simulink model "Pump_system_008"  (R2020a)
settings: Solver=VariableStepAuto  StartTime=0.0  StopTime=1000  MaxStep=0.5  RelTol=1e-3  AbsTol=1e-4
libraries: subsea_lib x65, nesl_utility x44
(part 2 of 2)

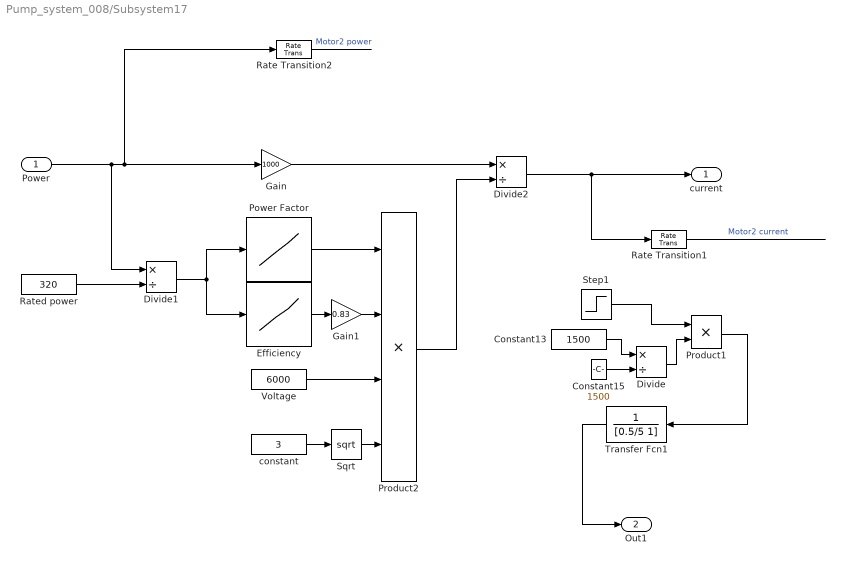
== system Pump_system_008/Subsystem17 ==
  Power : Inport
  Constant13 : Constant  Value=1500
  Constant15 : Constant  Value=1500
  Divide : Product  Inputs=*/
  Divide1 : Product  Inputs=*/
  Divide2 : Product  Inputs=*/
  Efficiency : Lookup_n-D  NumberOfTableDimensions=1  BreakpointsForDimension1=[0 0.05 0.25 0.5 0.75 1]  BreakpointsForDimension2=[1:3]  Table=[0 0.3 0.85 0.92 0.93 0.94]  InternalRulePriority=Speed  RndMeth=Simplest  InputSameDT=on
  Gain : Gain  Gain=1000
  Gain1 : Gain  Gain=0.83
  Power Factor : Lookup_n-D  NumberOfTableDimensions=1  BreakpointsForDimension1=[0 0.05 0.25 0.5 0.75 1]  BreakpointsForDimension2=[1:3]  Table=[0 0.3 0.7 0.83 0.85 0.87]  InternalRulePriority=Speed  RndMeth=Simplest  InputSameDT=on
  Product1 : Product
  Product2 : Product  Inputs=4
  Rate Transition1 : RateTransition  OutPortSampleTime=1
  Rate Transition2 : RateTransition  OutPortSampleTime=1
  Rated power : Constant  Value=320
  Sqrt : Sqrt  SaturateOnIntegerOverflow=on
  Step1 : Step  Time=0.1  SampleTime=0
  Transfer Fcn1 : TransferFcn  Denominator=[0.5/5 1]
  Voltage : Constant  Value=6000
  constant : Constant  Value=3
  current : Outport
  Out1 : Outport  Port=2
  wires:
  Gain/1 -> Divide2/1
  Product2/1 -> Divide2/2
  Power Factor/1 -> Product2/1
  Efficiency/1 -> Gain1/1
  Sqrt/1 -> Product2/4
  constant/1 -> Sqrt/1
  Voltage/1 -> Product2/3
  Divide1/1 -> Power Factor/1, Efficiency/1
  Rated power/1 -> Divide1/2
  Power/1 -> Rate Transition2/1, Gain/1, Divide1/1
  Step1/1 -> Product1/1
  Transfer Fcn1/1 -> Out1/1
  Constant15/1 -> Divide/2
  Divide/1 -> Product1/2
  Product1/1 -> Transfer Fcn1/1
  Constant13/1 -> Divide/1
  Rate Transition2/1 -> ?  "Motor2 power"
  Rate Transition1/1 -> ?  "Motor2 current"
  Divide2/1 -> Rate Transition1/1, current/1
  Gain1/1 -> Product2/2

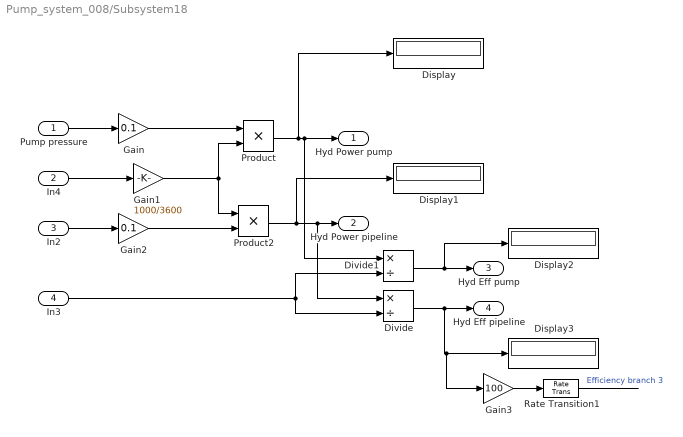
== system Pump_system_008/Subsystem18 ==
  Pump pressure : Inport
  In4 : Inport  Port=2
  In2 : Inport  Port=3
  In3 : Inport  Port=4
  Display{,1..3} (4 alike) : Display
      settings: Decimation=2
  Divide : Product  Inputs=*/
  Divide1 : Product  Inputs=*/
  Gain : Gain  Gain=0.1
  Gain1 : Gain  Gain=1000/3600
  Gain2 : Gain  Gain=0.1
  Gain3 : Gain  Gain=100
  Product : Product
  Product2 : Product
  Rate Transition1 : RateTransition  OutPortSampleTime=1
  Hyd Power pump : Outport
  Hyd Power pipeline : Outport  Port=2
  Hyd Eff pump : Outport  Port=3
  Hyd Eff pipeline : Outport  Port=4
  wires:
  Divide/1 -> Hyd Eff pipeline/1, Gain3/1, Display3/1
  Divide1/1 -> Hyd Eff pump/1, Display2/1
  Product2/1 -> Display1/1, Hyd Power pipeline/1, Divide/1
  Gain2/1 -> Product2/2
  Gain1/1 -> Product2/1, Product/2
  Gain/1 -> Product/1
  Pump pressure/1 -> Gain/1
  In3/1 -> Divide/2, Divide1/2
  In4/1 -> Gain1/1
  Product/1 -> Hyd Power pump/1, Divide1/1, Display/1
  In2/1 -> Gain2/1
  Gain3/1 -> Rate Transition1/1
  Rate Transition1/1 -> ?  "Efficiency branch 3"

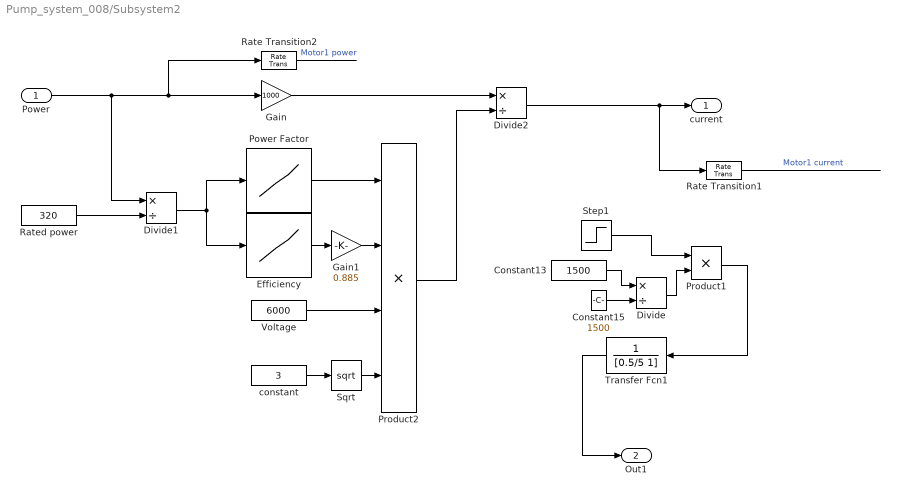
== system Pump_system_008/Subsystem2 ==
  Power : Inport
  Constant13 : Constant  Value=1500
  Constant15 : Constant  Value=1500
  Divide : Product  Inputs=*/
  Divide1 : Product  Inputs=*/
  Divide2 : Product  Inputs=*/
  Efficiency : Lookup_n-D  NumberOfTableDimensions=1  BreakpointsForDimension1=[0 0.05 0.25 0.5 0.75 1]  BreakpointsForDimension2=[1:3]  Table=[0 0.3 0.85 0.92 0.93 0.94]  InternalRulePriority=Speed  RndMeth=Simplest  InputSameDT=on
  Gain : Gain  Gain=1000
  Gain1 : Gain  Gain=0.885
  Power Factor : Lookup_n-D  NumberOfTableDimensions=1  BreakpointsForDimension1=[0 0.05 0.25 0.5 0.75 1]  BreakpointsForDimension2=[1:3]  Table=[0 0.3 0.7 0.85 0.88 0.92]  InternalRulePriority=Speed  RndMeth=Simplest  InputSameDT=on
  Product1 : Product
  Product2 : Product  Inputs=4
  Rate Transition1 : RateTransition  OutPortSampleTime=1
  Rate Transition2 : RateTransition  OutPortSampleTime=1
  Rated power : Constant  Value=320
  Sqrt : Sqrt  SaturateOnIntegerOverflow=on
  Step1 : Step  Time=0.1  SampleTime=0
  Transfer Fcn1 : TransferFcn  Denominator=[0.5/5 1]
  Voltage : Constant  Value=6000
  constant : Constant  Value=3
  current : Outport
  Out1 : Outport  Port=2
  wires:
  Constant13/1 -> Divide/1
  Product1/1 -> Transfer Fcn1/1
  Divide/1 -> Product1/2
  Constant15/1 -> Divide/2
  Transfer Fcn1/1 -> Out1/1
  Step1/1 -> Product1/1
  Power/1 -> Divide1/1, Rate Transition2/1, Gain/1
  Rated power/1 -> Divide1/2
  Divide1/1 -> Efficiency/1, Power Factor/1
  Voltage/1 -> Product2/3
  constant/1 -> Sqrt/1
  Sqrt/1 -> Product2/4
  Efficiency/1 -> Gain1/1
  Power Factor/1 -> Product2/1
  Product2/1 -> Divide2/2
  Gain/1 -> Divide2/1
  Divide2/1 -> Rate Transition1/1, current/1
  Rate Transition1/1 -> ?  "Motor1 current"
  Rate Transition2/1 -> ?  "Motor1 power"
  Gain1/1 -> Product2/2

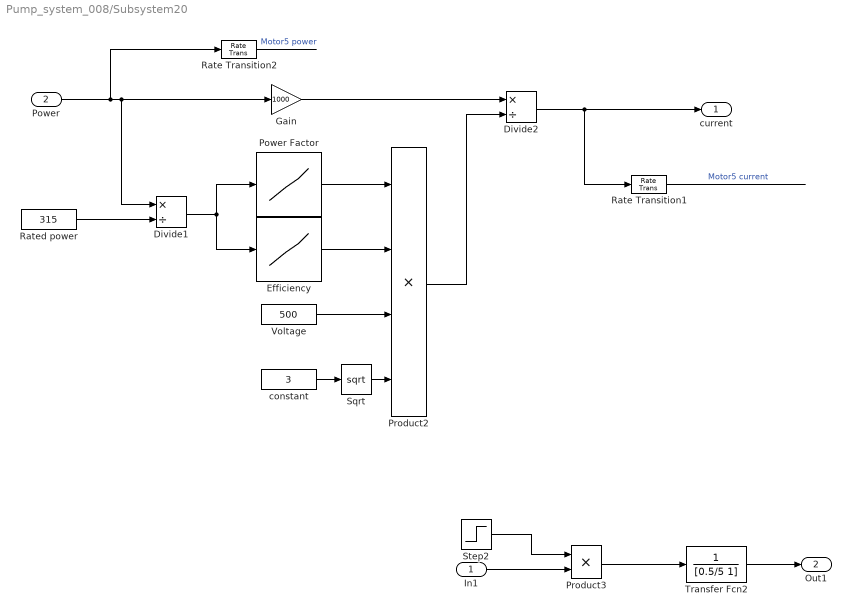
== system Pump_system_008/Subsystem20 ==
  In1 : Inport
  Power : Inport  Port=2
  Divide1 : Product  Inputs=*/
  Divide2 : Product  Inputs=*/
  Efficiency : Lookup_n-D  NumberOfTableDimensions=1  BreakpointsForDimension1=[0 0.05 0.25 0.5 0.75 1]  BreakpointsForDimension2=[1:3]  Table=[0 0.3 0.85 0.956 0.96 0.959]  InternalRulePriority=Speed  RndMeth=Simplest  InputSameDT=on
  Gain : Gain  Gain=1000
  Power Factor : Lookup_n-D  NumberOfTableDimensions=1  BreakpointsForDimension1=[0 0.05 0.25 0.5 0.75 1]  BreakpointsForDimension2=[1:3]  Table=[0 0.85 0.97 0.975 0.978 0.98]  InternalRulePriority=Speed  RndMeth=Simplest  InputSameDT=on
  Product2 : Product  Inputs=4
  Product3 : Product
  Rate Transition1 : RateTransition  OutPortSampleTime=1
  Rate Transition2 : RateTransition  OutPortSampleTime=1
  Rated power : Constant  Value=315
  Sqrt : Sqrt  SaturateOnIntegerOverflow=on
  Step2 : Step  Time=0.1  SampleTime=0
  Transfer Fcn2 : TransferFcn  Denominator=[0.5/5 1]
  Voltage : Constant  Value=500
  constant : Constant  Value=3
  current : Outport
  Out1 : Outport  Port=2
  wires:
  Transfer Fcn2/1 -> Out1/1
  In1/1 -> Product3/2
  Step2/1 -> Product3/1
  Product3/1 -> Transfer Fcn2/1
  Gain/1 -> Divide2/1
  Product2/1 -> Divide2/2
  Power Factor/1 -> Product2/1
  Efficiency/1 -> Product2/2
  Sqrt/1 -> Product2/4
  constant/1 -> Sqrt/1
  Voltage/1 -> Product2/3
  Divide1/1 -> Power Factor/1, Efficiency/1
  Rated power/1 -> Divide1/2
  Rate Transition2/1 -> ?  "Motor5 power"
  Power/1 -> Rate Transition2/1, Gain/1, Divide1/1
  Rate Transition1/1 -> ?  "Motor5 current"
  Divide2/1 -> Rate Transition1/1, current/1

== system Pump_system_008/Subsystem21 ==
  Pump p : Inport
  RPM : Inport  Port=2
  Pump : Subsystem
  Subsea Hydraulic Flow Source : subsea_lib/Sources/Subsea Hydraulic Flow Source
      settings: SourceProductName=Subsea  InternalSimscapePortConfiguration="{\"Bottom\":[],\"Left\":[{\"id\":\"P\",\"label\":\"P\",\"type\":\"subsea.ss_hydraulic\"}],\"Right\":[{\"id\":\"S\",\"label\":\"S\",\"type\":\"input\"},{\"id\":\"T\",\"label\":\"T\",\"type\":\"subsea.ss_hydraulic\"}],\"Top\":[]}"
  Subsea Hydraulic Flow Source2 : PMIOPort  Side=Left
  Subsea Hydraulic Flow Source1 : PMIOPort  Port=2  Side=Right
  Power : Outport
  wires:
  Pump p/1 -> Pump/2(Pump p)
  RPM/1 -> Pump/1(RPM)
  Pump/1(Power) -> Power/1
  connections:
  Subsea Hydraulic Flow Source/RConn1 -- Pump/RConn1
  Subsea Hydraulic Flow Source/RConn2 -- Subsea Hydraulic Flow Source2/RConn1
  Subsea Hydraulic Flow Source/LConn1 -- Subsea Hydraulic Flow Source1/RConn1

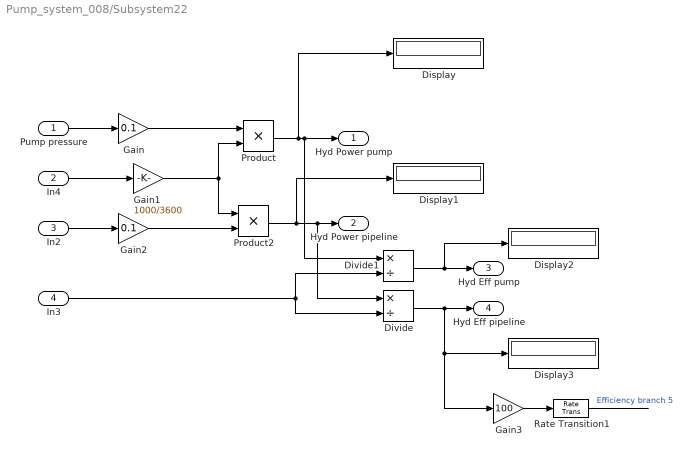
== system Pump_system_008/Subsystem22 ==
  Pump pressure : Inport
  In4 : Inport  Port=2
  In2 : Inport  Port=3
  In3 : Inport  Port=4
  Display{,1..3} (4 alike) : Display
      settings: Decimation=2
  Divide : Product  Inputs=*/
  Divide1 : Product  Inputs=*/
  Gain : Gain  Gain=0.1
  Gain1 : Gain  Gain=1000/3600
  Gain2 : Gain  Gain=0.1
  Gain3 : Gain  Gain=100
  Product : Product
  Product2 : Product
  Rate Transition1 : RateTransition  OutPortSampleTime=1
  Hyd Power pump : Outport
  Hyd Power pipeline : Outport  Port=2
  Hyd Eff pump : Outport  Port=3
  Hyd Eff pipeline : Outport  Port=4
  wires:
  Divide1/1 -> Hyd Eff pump/1, Display2/1
  Product2/1 -> Display1/1, Hyd Power pipeline/1, Divide/1
  Gain2/1 -> Product2/2
  Gain1/1 -> Product2/1, Product/2
  Gain/1 -> Product/1
  Pump pressure/1 -> Gain/1
  In3/1 -> Divide/2, Divide1/2
  In4/1 -> Gain1/1
  Product/1 -> Hyd Power pump/1, Divide1/1, Display/1
  In2/1 -> Gain2/1
  Gain3/1 -> Rate Transition1/1
  Rate Transition1/1 -> ?  "Efficiency branch 5"
  Divide/1 -> Hyd Eff pipeline/1, Gain3/1, Display3/1

== system Pump_system_008/Subsystem23 ==
  Gain : Gain  Gain=3600
  PS-Simulink Converter5 : nesl_utility/PS-Simulink Converter  PhysicalDomain=network_engine_domain  SubClassName=ps_output  LeftPortType=input  RightPortType=output  PseudoPeriodic=off  Frequencies=[]  Unit=m^3/s  AffineConversion=off
      settings: SourceProductBaseCode=MT,SS
  in : PMIOPort  Side=Left
  Q m3/h : Outport
  wires:
  PS-Simulink Converter5/1 -> Gain/1
  Gain/1 -> Q m3/h/1
  connections:
  PS-Simulink Converter5/LConn1 -- in/RConn1

== system Pump_system_008/Subsystem24 ==
  Gain : Gain  Gain=3600
  PS-Simulink Converter5 : nesl_utility/PS-Simulink Converter  PhysicalDomain=network_engine_domain  SubClassName=ps_output  LeftPortType=input  RightPortType=output  PseudoPeriodic=off  Frequencies=[]  Unit=m^3/s  AffineConversion=off
      settings: SourceProductBaseCode=MT,SS
  in : PMIOPort  Side=Left
  Q m3/h : Outport
  wires:
  PS-Simulink Converter5/1 -> Gain/1
  Gain/1 -> Q m3/h/1
  connections:
  PS-Simulink Converter5/LConn1 -- in/RConn1

== system Pump_system_008/Subsystem25 ==
  Pump p : Inport
  RPM : Inport  Port=2
  Pump : Subsystem
  Subsea Hydraulic Flow Source : subsea_lib/Sources/Subsea Hydraulic Flow Source
      settings: SourceProductName=Subsea  InternalSimscapePortConfiguration="{\"Bottom\":[],\"Left\":[{\"id\":\"P\",\"label\":\"P\",\"type\":\"subsea.ss_hydraulic\"}],\"Right\":[{\"id\":\"S\",\"label\":\"S\",\"type\":\"input\"},{\"id\":\"T\",\"label\":\"T\",\"type\":\"subsea.ss_hydraulic\"}],\"Top\":[]}"
  Subsea Hydraulic Flow Source2 : PMIOPort  Side=Left
  Subsea Hydraulic Flow Source1 : PMIOPort  Port=2  Side=Right
  Power : Outport
  wires:
  Pump/1(Power) -> Power/1
  RPM/1 -> Pump/1(RPM)
  Pump p/1 -> Pump/2(Pump p)
  connections:
  Subsea Hydraulic Flow Source/LConn1 -- Subsea Hydraulic Flow Source1/RConn1
  Subsea Hydraulic Flow Source/RConn2 -- Subsea Hydraulic Flow Source2/RConn1
  Subsea Hydraulic Flow Source/RConn1 -- Pump/RConn1

== system Pump_system_008/Subsystem26 ==
  In1 : Inport
  Product1 : Product
  Step1 : Step  Time=0.1  SampleTime=0
  Transfer Fcn1 : TransferFcn  Denominator=[0.5/5 1]
  Out1 : Outport
  wires:
  Step1/1 -> Product1/1
  Transfer Fcn1/1 -> Out1/1
  In1/1 -> Product1/2
  Product1/1 -> Transfer Fcn1/1

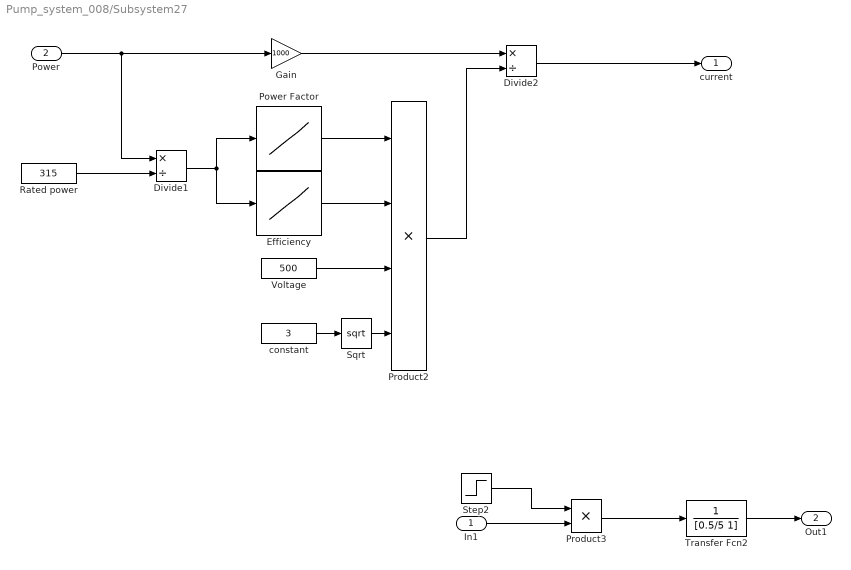
== system Pump_system_008/Subsystem27 ==
  In1 : Inport
  Power : Inport  Port=2
  Divide1 : Product  Inputs=*/
  Divide2 : Product  Inputs=*/
  Efficiency : Lookup_n-D  NumberOfTableDimensions=1  BreakpointsForDimension1=[0 0.05 0.25 0.5 0.75 1]  BreakpointsForDimension2=[1:3]  Table=[0 0.3 0.85 0.956 0.96 0.959]  InternalRulePriority=Speed  RndMeth=Simplest  InputSameDT=on
  Gain : Gain  Gain=1000
  Power Factor : Lookup_n-D  NumberOfTableDimensions=1  BreakpointsForDimension1=[0 0.05 0.25 0.5 0.75 1]  BreakpointsForDimension2=[1:3]  Table=[0 0.3 0.7 0.8 0.88 0.9]  InternalRulePriority=Speed  RndMeth=Simplest  InputSameDT=on
  Product2 : Product  Inputs=4
  Product3 : Product
  Rated power : Constant  Value=315
  Sqrt : Sqrt  SaturateOnIntegerOverflow=on
  Step2 : Step  Time=0.1  SampleTime=0
  Transfer Fcn2 : TransferFcn  Denominator=[0.5/5 1]
  Voltage : Constant  Value=500
  constant : Constant  Value=3
  current : Outport
  Out1 : Outport  Port=2
  wires:
  Power/1 -> Divide1/1, Gain/1
  Rated power/1 -> Divide1/2
  Divide1/1 -> Efficiency/1, Power Factor/1
  Voltage/1 -> Product2/3
  constant/1 -> Sqrt/1
  Sqrt/1 -> Product2/4
  Efficiency/1 -> Product2/2
  Power Factor/1 -> Product2/1
  Product2/1 -> Divide2/2
  Gain/1 -> Divide2/1
  Divide2/1 -> current/1
  Product3/1 -> Transfer Fcn2/1
  Step2/1 -> Product3/1
  In1/1 -> Product3/2
  Transfer Fcn2/1 -> Out1/1

== system Pump_system_008/Subsystem3 ==
  Gain : Gain  Gain=3600
  PS-Simulink Converter5 : nesl_utility/PS-Simulink Converter  PhysicalDomain=network_engine_domain  SubClassName=ps_output  LeftPortType=input  RightPortType=output  PseudoPeriodic=off  Frequencies=[]  Unit=m^3/s  AffineConversion=off
      settings: SourceProductBaseCode=MT,SS
  in : PMIOPort  Side=Left
  Q m3/h : Outport
  wires:
  Gain/1 -> Q m3/h/1
  PS-Simulink Converter5/1 -> Gain/1
  connections:
  PS-Simulink Converter5/LConn1 -- in/RConn1

== system Pump_system_008/Subsystem4 ==
  Gain : Gain  Gain=3600
  PS-Simulink Converter5 : nesl_utility/PS-Simulink Converter  PhysicalDomain=network_engine_domain  SubClassName=ps_output  LeftPortType=input  RightPortType=output  PseudoPeriodic=off  Frequencies=[]  Unit=m^3/s  AffineConversion=off
      settings: SourceProductBaseCode=MT,SS
  in : PMIOPort  Side=Left
  Q m3/h : Outport
  wires:
  PS-Simulink Converter5/1 -> Gain/1
  Gain/1 -> Q m3/h/1
  connections:
  PS-Simulink Converter5/LConn1 -- in/RConn1

== system Pump_system_008/Subsystem5 ==
  Pump p : Inport
  RPM : Inport  Port=2
  Pump : Subsystem
  Subsea Hydraulic Flow Source : subsea_lib/Sources/Subsea Hydraulic Flow Source
      settings: SourceProductName=Subsea  InternalSimscapePortConfiguration="{\"Bottom\":[],\"Left\":[{\"id\":\"P\",\"label\":\"P\",\"type\":\"subsea.ss_hydraulic\"}],\"Right\":[{\"id\":\"S\",\"label\":\"S\",\"type\":\"input\"},{\"id\":\"T\",\"label\":\"T\",\"type\":\"subsea.ss_hydraulic\"}],\"Top\":[]}"
  Subsea Hydraulic Flow Source2 : PMIOPort  Side=Left
  Subsea Hydraulic Flow Source1 : PMIOPort  Port=2  Side=Right
  Power : Outport
  wires:
  Pump/1(Power) -> Power/1
  RPM/1 -> Pump/1(RPM)
  Pump p/1 -> Pump/2(Pump p)
  connections:
  Subsea Hydraulic Flow Source/LConn1 -- Subsea Hydraulic Flow Source1/RConn1
  Subsea Hydraulic Flow Source/RConn2 -- Subsea Hydraulic Flow Source2/RConn1
  Subsea Hydraulic Flow Source/RConn1 -- Pump/RConn1

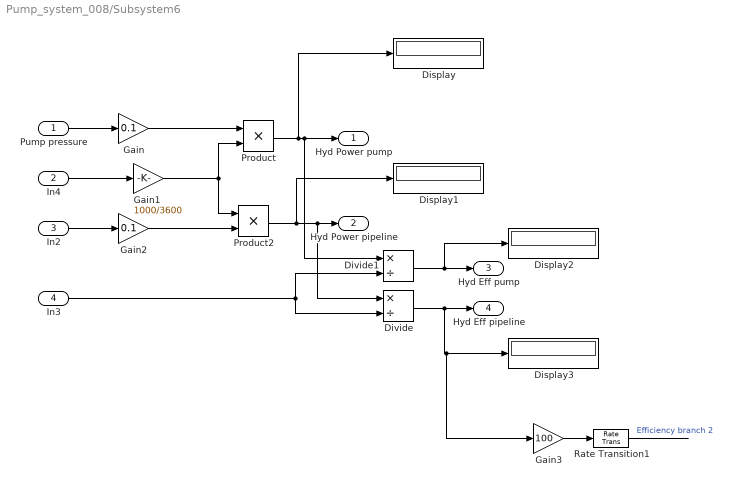
== system Pump_system_008/Subsystem6 ==
  Pump pressure : Inport
  In4 : Inport  Port=2
  In2 : Inport  Port=3
  In3 : Inport  Port=4
  Display{,1..3} (4 alike) : Display
      settings: Decimation=2
  Divide : Product  Inputs=*/
  Divide1 : Product  Inputs=*/
  Gain : Gain  Gain=0.1
  Gain1 : Gain  Gain=1000/3600
  Gain2 : Gain  Gain=0.1
  Gain3 : Gain  Gain=100
  Product : Product
  Product2 : Product
  Rate Transition1 : RateTransition  OutPortSampleTime=1
  Hyd Power pump : Outport
  Hyd Power pipeline : Outport  Port=2
  Hyd Eff pump : Outport  Port=3
  Hyd Eff pipeline : Outport  Port=4
  wires:
  Divide/1 -> Hyd Eff pipeline/1, Gain3/1, Display3/1
  Divide1/1 -> Hyd Eff pump/1, Display2/1
  Product2/1 -> Display1/1, Hyd Power pipeline/1, Divide/1
  Gain2/1 -> Product2/2
  Gain1/1 -> Product2/1, Product/2
  Gain/1 -> Product/1
  Pump pressure/1 -> Gain/1
  In3/1 -> Divide/2, Divide1/2
  In4/1 -> Gain1/1
  Product/1 -> Hyd Power pump/1, Divide1/1, Display/1
  In2/1 -> Gain2/1
  Gain3/1 -> Rate Transition1/1
  Rate Transition1/1 -> ?  "Efficiency branch 2"

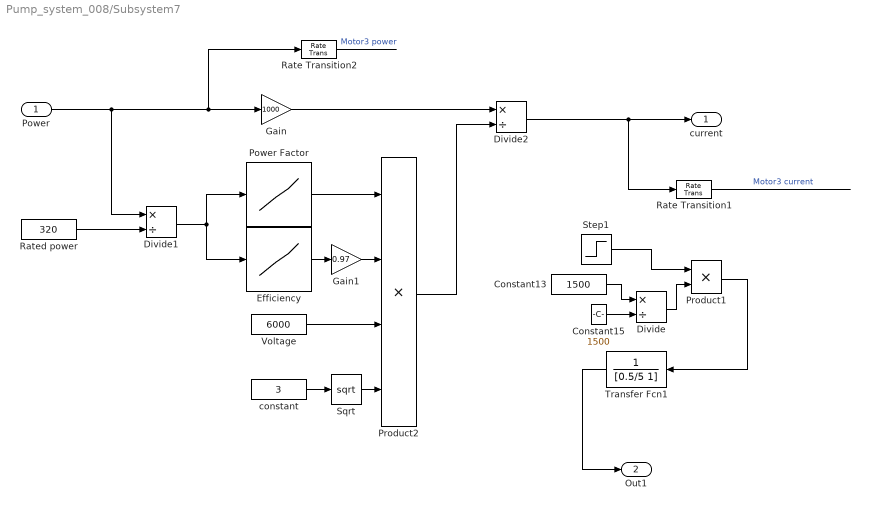
== system Pump_system_008/Subsystem7 ==
  Power : Inport
  Constant13 : Constant  Value=1500
  Constant15 : Constant  Value=1500
  Divide : Product  Inputs=*/
  Divide1 : Product  Inputs=*/
  Divide2 : Product  Inputs=*/
  Efficiency : Lookup_n-D  NumberOfTableDimensions=1  BreakpointsForDimension1=[0 0.05 0.25 0.5 0.75 1]  BreakpointsForDimension2=[1:3]  Table=[0 0.3 0.85 0.92 0.93 0.94]  InternalRulePriority=Speed  RndMeth=Simplest  InputSameDT=on
  Gain : Gain  Gain=1000
  Gain1 : Gain  Gain=0.97
  Power Factor : Lookup_n-D  NumberOfTableDimensions=1  BreakpointsForDimension1=[0 0.05 0.25 0.5 0.75 1]  BreakpointsForDimension2=[1:3]  Table=[0 0.3 0.7 0.83 0.85 0.87]  InternalRulePriority=Speed  RndMeth=Simplest  InputSameDT=on
  Product1 : Product
  Product2 : Product  Inputs=4
  Rate Transition1 : RateTransition  OutPortSampleTime=1
  Rate Transition2 : RateTransition  OutPortSampleTime=1
  Rated power : Constant  Value=320
  Sqrt : Sqrt  SaturateOnIntegerOverflow=on
  Step1 : Step  Time=0.1  SampleTime=0
  Transfer Fcn1 : TransferFcn  Denominator=[0.5/5 1]
  Voltage : Constant  Value=6000
  constant : Constant  Value=3
  current : Outport
  Out1 : Outport  Port=2
  wires:
  Gain/1 -> Divide2/1
  Product2/1 -> Divide2/2
  Power Factor/1 -> Product2/1
  Efficiency/1 -> Gain1/1
  Sqrt/1 -> Product2/4
  constant/1 -> Sqrt/1
  Voltage/1 -> Product2/3
  Divide1/1 -> Power Factor/1, Efficiency/1
  Rated power/1 -> Divide1/2
  Step1/1 -> Product1/1
  Transfer Fcn1/1 -> Out1/1
  Constant15/1 -> Divide/2
  Divide/1 -> Product1/2
  Product1/1 -> Transfer Fcn1/1
  Constant13/1 -> Divide/1
  Rate Transition2/1 -> ?  "Motor3 power"
  Power/1 -> Rate Transition2/1, Gain/1, Divide1/1
  Rate Transition1/1 -> ?  "Motor3 current"
  Divide2/1 -> Rate Transition1/1, current/1
  Gain1/1 -> Product2/2

== system Pump_system_008/Subsystem8 ==
  Gain : Gain  Gain=3600
  PS-Simulink Converter5 : nesl_utility/PS-Simulink Converter  PhysicalDomain=network_engine_domain  SubClassName=ps_output  LeftPortType=input  RightPortType=output  PseudoPeriodic=off  Frequencies=[]  Unit=m^3/s  AffineConversion=off
      settings: SourceProductBaseCode=MT,SS
  in : PMIOPort  Side=Left
  Q m3/h : Outport
  wires:
  PS-Simulink Converter5/1 -> Gain/1
  Gain/1 -> Q m3/h/1
  connections:
  PS-Simulink Converter5/LConn1 -- in/RConn1

== system Pump_system_008/Subsystem9 ==
  Pump p : Inport
  RPM : Inport  Port=2
  Pump : Subsystem
  Subsea Hydraulic Flow Source : subsea_lib/Sources/Subsea Hydraulic Flow Source
      settings: SourceProductName=Subsea  InternalSimscapePortConfiguration="{\"Bottom\":[],\"Left\":[{\"id\":\"P\",\"label\":\"P\",\"type\":\"subsea.ss_hydraulic\"}],\"Right\":[{\"id\":\"S\",\"label\":\"S\",\"type\":\"input\"},{\"id\":\"T\",\"label\":\"T\",\"type\":\"subsea.ss_hydraulic\"}],\"Top\":[]}"
  Subsea Hydraulic Flow Source2 : PMIOPort  Side=Left
  Subsea Hydraulic Flow Source1 : PMIOPort  Port=2  Side=Right
  Power : Outport
  wires:
  Pump/1(Power) -> Power/1
  RPM/1 -> Pump/1(RPM)
  Pump p/1 -> Pump/2(Pump p)
  connections:
  Subsea Hydraulic Flow Source/LConn1 -- Subsea Hydraulic Flow Source1/RConn1
  Subsea Hydraulic Flow Source/RConn2 -- Subsea Hydraulic Flow Source2/RConn1
  Subsea Hydraulic Flow Source/RConn1 -- Pump/RConn1

== system Pump_system_008/Tank ==
  Custom Hydraulic Fluid1 : subsea_lib/Environment Elements/Custom Hydraulic Fluid  density=1000 kg/m^3  sea_density=1025 kg/m^3  viscosity_kin=0.89 cSt  viscosity_subsea=0.89 cSt  viscosity_topside=0.89 cSt  bulk=2800 MPa  alpha=0.005  depth=0 m  rig_elev=0 m  range_error=2
      settings: SourceProductName=Subsea  InternalSimscapePortConfiguration="{\"Bottom\":[],\"Left\":[],\"Right\":[{\"id\":\"G\",\"label\":\"\",\"type\":\"subsea.ss_hydraulic\"}],\"Top\":[]}"
  Solver Configuration1 : nesl_utility/Solver Configuration  PhysicalDomain=network_engine_domain  SubClassName=solver  LeftPortType=input  RightPortType=generic  Tones=[]  Harmonics=[]  SimulateNoise=off  Profile=off  UseLocalSampling=off  EnableSwitchedLinearOptims=on  FrequencyDomain=off  UseCCode=off  RelTol=0.001  AbsTol=1e-06  MinStep=1e-09  ToWorkspace=off  RevertToSquareIcSolve=off  NumHomotopyIterations=100  PhasorMode=off  PhasorModeNumHarmonics=1  DoDC=off  ResidualTolerance=1e-05  UseLocalSolver=off  LocalSolverChoice=NE_BACKWARD_EULER_ADVANCER  LocalSolverSampleTime=0.001  DoFixedCost=off  MaxNonlinIter=3  MaxModeIter=2  LinearAlgebra=auto  EquationFormulation=NE_TIME_EF  DelaysMemoryBudget=1024  AutomaticFiltering=on  FilteringTimeConstant=0.001  PartitionStorageMethod=AS_NEEDED  PartitionMemoryBudget=1024  PartitionMethod=ROBUST
  Subsea Hydraulic Reference2 : subsea_lib/Environment Elements/Subsea Hydraulic Reference
      settings: SourceProductName=Subsea  InternalSimscapePortConfiguration="{\"Bottom\":[],\"Left\":[{\"id\":\"P\",\"label\":\"\",\"type\":\"subsea.ss_hydraulic\"}],\"Right\":[],\"Top\":[]}"
  Conn1 : PMIOPort  Side=Left
  connections:
  Solver Configuration1/RConn1 -- Conn1/RConn1 -- Custom Hydraulic Fluid1/RConn1 -- Subsea Hydraulic Reference2/LConn1

== system Pump_system_008/restriction ==
  In1 : Inport
  Simulink-PS Converter4 : nesl_utility/Simulink-PS Converter  PhysicalDomain=network_engine_domain  SubClassName=ps_input  LeftPortType=input  RightPortType=output  PseudoPeriodic=off  Frequencies=[]  NoiseDistribution=none  NoiseParameters=[]  Unit=m^3/s  AffineConversion=off  FilteringAndDerivatives=provide  SimscapeFilterOrder=1  InputFilterTimeConstant=0.001  UdotUserProvided=0
      settings: SourceProductBaseCode=MT,SS
  Variable kv Hydraulic Flow Element : subsea_lib/Valves/Variable kv Hydraulic Flow Element  ss_location=true  kv=1/3600 m^3/s  kv_min=1.3e-6 m^3/s  q_specify=off  q_priority=None  q=0 m^3/s  q_nominal_specify=off  q_nominal_unit=m^3/s  q_nominal_value=1  p_specify=off  p_priority=None  p=0 Pa  p_nominal_specify=off  p_nominal_unit=Pa  p_nominal_value=1
      settings: SourceProductName=Subsea  InternalSimscapePortConfiguration="{\"Bottom\":[],\"Left\":[{\"id\":\"CS\",\"label\":\"CS\",\"type\":\"input\"},{\"id\":\"A\",\"label\":\"A\",\"type\":\"subsea.ss_hydraulic\"}],\"Right\":[{\"id\":\"B\",\"label\":\"B\",\"type\":\"subsea.ss_hydraulic\"}],\"Top\":[]}"
  buterfly : Lookup_n-D  NumberOfTableDimensions=1  BreakpointsForDimension1=[0 45 90]  BreakpointsForDimension2=[1:3]  Table=[0 900 1800]  InternalRulePriority=Speed  RndMeth=Simplest  InputSameDT=on
  Variable kv Hydraulic Flow Element1 : PMIOPort  Side=Left
  Variable kv Hydraulic Flow Element2 : PMIOPort  Port=2  Side=Right
  wires:
  In1/1 -> buterfly/1
  buterfly/1 -> Simulink-PS Converter4/1
  connections:
  Variable kv Hydraulic Flow Element/LConn2 -- Variable kv Hydraulic Flow Element1/RConn1
  Simulink-PS Converter4/RConn1 -- Variable kv Hydraulic Flow Element/LConn1
  Variable kv Hydraulic Flow Element/RConn1 -- Variable kv Hydraulic Flow Element2/RConn1

== system Pump_system_008/Subsystem12/Pump ==
  RPM : Inport
  Pump p : Inport  Port=2
  Gain : Gain  Gain=1/3600
  Power and Flow : Scope  NumInputPorts=2
  Product1 : Product
  Pump characteristic : Lookup_n-D  NumberOfTableDimensions=1  BreakpointsForDimension1=[0,4.4,5.6,7.2,7.8,8.4,8.8,9.3,9.7,10,10.2,10.3,10.35,10.351,10.352]  Table=[1600,1375,1200,1000,900,800,700,600,500,400,300,200,175,100,0]  InterpMethod=Akima spline  InternalRulePriority=Speed  RndMeth=Simplest  InputSameDT=on
  Pump efficiency : Lookup_n-D  NumberOfTableDimensions=1  BreakpointsForDimension1=[0,100,200,300,400,500,600,700,800,900,1000,1075,1200,1300,1375,1600]  Table=[2,15,26,37,46,55,62,67,71,74,75,76,74.5,72,70,50]  InterpMethod=Akima spline  InternalRulePriority=Speed  RndMeth=Simplest  InputSameDT=on
  Rate Transition1 : RateTransition  OutPortSampleTime=1
  Rate Transition12 : RateTransition  OutPortSampleTime=1
  Rate Transition2 : RateTransition  OutPortSampleTime=1
  Simulink-PS Converter1 : nesl_utility/Simulink-PS Converter  PhysicalDomain=network_engine_domain  SubClassName=ps_input  LeftPortType=input  RightPortType=output  PseudoPeriodic=off  Frequencies=[]  NoiseDistribution=none  NoiseParameters=[]  Unit=m^3/s  AffineConversion=off  FilteringAndDerivatives=provide  SimscapeFilterOrder=1  InputFilterTimeConstant=0.001  UdotUserProvided=0
      settings: SourceProductBaseCode=MT,SS
  Subsystem : Subsystem
  output : PMIOPort  Side=Right
  Power : Outport
  wires:
  RPM/1 -> Product1/1  "RPM"
  Pump characteristic/1 -> Pump efficiency/1, Product1/2
  Pump p/1 -> Rate Transition1/1, Pump characteristic/1, Subsystem/3(p)
  Subsystem/1(Power) -> Rate Transition12/1, Power/1, Power and Flow/2  "Power"
  Pump efficiency/1 -> Subsystem/2(eff)
  Rate Transition12/1 -> ?  "Pump1 power"
  Rate Transition1/1 -> ?  "Pump1 pressure"
  Rate Transition2/1 -> ?  "Pump1 flow"
  Product1/1 -> Rate Transition2/1, Power and Flow/1, Gain/1
  Gain/1 -> Simulink-PS Converter1/1, Subsystem/1(flow)
  connections:
  output/RConn1 -- Simulink-PS Converter1/RConn1

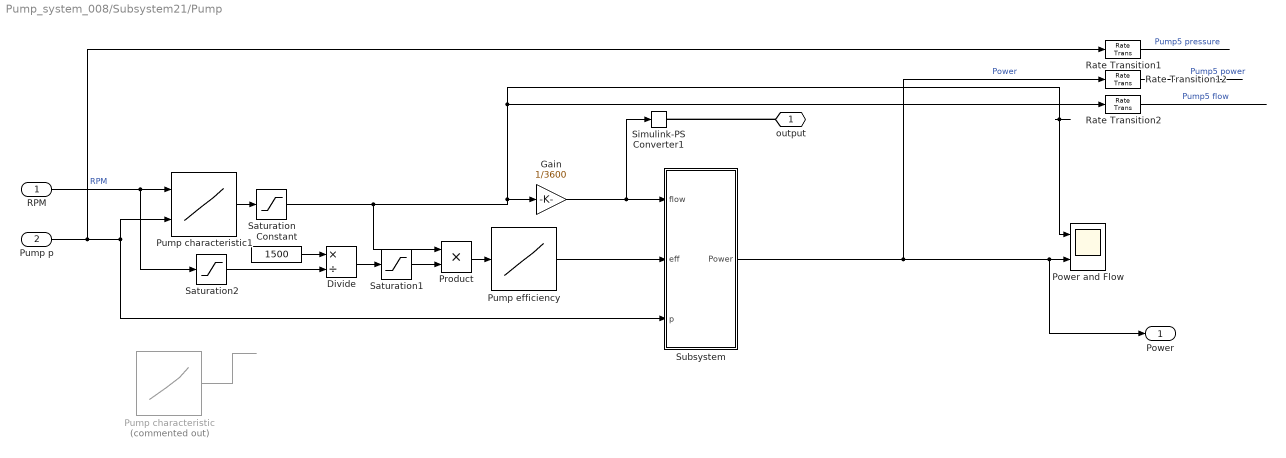
== system Pump_system_008/Subsystem21/Pump ==
  RPM : Inport
  Pump p : Inport  Port=2
  Constant : Constant  Value=1500
  Divide : Product  Inputs=*/
  Gain : Gain  Gain=1/3600
  Power and Flow : Scope  NumInputPorts=2
  Product : Product
  Pump characteristic : Lookup_n-D  Commented=on  NumberOfTableDimensions=1  BreakpointsForDimension1=[0,4.4,5.6,7.2,7.8,8.4,8.8,9.3,9.7,10,10.2,10.3,10.35,10.351,10.352]  Table=[1600,1375,1200,1000,900,800,700,600,500,400,300,200,175,100,0]  InterpMethod=Akima spline  InternalRulePriority=Speed  RndMeth=Simplest  InputSameDT=on
  Pump characteristic1 : Lookup_n-D  BreakpointsForDimension1=[1000,1200,1400,1500]  BreakpointsForDimension2=[0,4.4,5.6,7.2,7.8,8.4,8.8,9.3,9.7,10,10.2,10.3,10.35,10.351,10.352]  Table=reshape([1066,1280,1493,1600,719,971,1249,1375,533,822,1073,1200,0,527.5,853.5,1000,0,388.5,754.4,900,0,5,615.3,800,0,0,532.3,700,0,0,385.6,600,0,0,5,500,0,0,0,400,0,0,0,300,0,0,0,200,0,0,0,175,0,0,0,100,0,0,0,0],4,15)  InterpMethod=Akima spline  InternalRulePriority=Speed  RndMeth=Simplest  InputSameDT=on
  Pump efficiency : Lookup_n-D  NumberOfTableDimensions=1  BreakpointsForDimension1=[0,100,200,300,400,500,600,700,800,900,1000,1075,1200,1300,1375,1600]  Table=[2,15,26,37,46,55,62,67,71,74,75,76,74.5,72,70,50]  InterpMethod=Akima spline  InternalRulePriority=Speed  RndMeth=Simplest  InputSameDT=on
  Rate Transition1 : RateTransition  OutPortSampleTime=1
  Rate Transition12 : RateTransition  OutPortSampleTime=1
  Rate Transition2 : RateTransition  OutPortSampleTime=1
  Saturation : Saturate  UpperLimit=inf  LowerLimit=0
  Saturation1 : Saturate  UpperLimit=2  LowerLimit=0
  Saturation2 : Saturate  UpperLimit=inf  LowerLimit=1
  Simulink-PS Converter1 : nesl_utility/Simulink-PS Converter  PhysicalDomain=network_engine_domain  SubClassName=ps_input  LeftPortType=input  RightPortType=output  PseudoPeriodic=off  Frequencies=[]  NoiseDistribution=none  NoiseParameters=[]  Unit=m^3/s  AffineConversion=off  FilteringAndDerivatives=provide  SimscapeFilterOrder=1  InputFilterTimeConstant=0.001  UdotUserProvided=0
      settings: SourceProductBaseCode=MT,SS
  Subsystem : Subsystem
  output : PMIOPort  Side=Right
  Power : Outport
  wires:
  Saturation/1 -> Product/1, Rate Transition2/1, Power and Flow/1, Gain/1
  Pump p/1 -> Rate Transition1/1, Subsystem/3(p), Pump characteristic1/2
  Pump characteristic/1 -> ?
  RPM/1 -> Saturation2/1, Pump characteristic1/1  "RPM"
  Subsystem/1(Power) -> Rate Transition12/1, Power/1, Power and Flow/2  "Power"
  Pump efficiency/1 -> Subsystem/2(eff)
  Pump characteristic1/1 -> Saturation/1
  Gain/1 -> Simulink-PS Converter1/1, Subsystem/1(flow)
  Constant/1 -> Divide/1
  Divide/1 -> Saturation1/1
  Product/1 -> Pump efficiency/1
  Saturation1/1 -> Product/2
  Saturation2/1 -> Divide/2
  Rate Transition2/1 -> ?  "Pump5 flow"
  Rate Transition1/1 -> ?  "Pump5 pressure"
  Rate Transition12/1 -> ?  "Pump5 power"
  connections:
  output/RConn1 -- Simulink-PS Converter1/RConn1

== system Pump_system_008/Subsystem25/Pump ==
  RPM : Inport
  Pump p : Inport  Port=2
  Gain : Gain  Gain=1/3600
  Power and Flow : Scope  NumInputPorts=2
  Pump characteristic : Lookup_n-D  Commented=on  NumberOfTableDimensions=1  BreakpointsForDimension1=[0,4.4,5.6,7.2,7.8,8.4,8.8,9.3,9.7,10,10.2,10.3,10.35,10.351,10.352]  Table=[1600,1375,1200,1000,900,800,700,600,500,400,300,200,175,100,0]  InterpMethod=Akima spline  InternalRulePriority=Speed  RndMeth=Simplest  InputSameDT=on
  Pump characteristic1 : Lookup_n-D  BreakpointsForDimension1=[1000,1200,1400,1500]  BreakpointsForDimension2=[0,4.4,5.6,7.2,7.8,8.4,8.8,9.3,9.7,10,10.2,10.3,10.35,10.351,10.352]  Table=reshape([1066,1280,1493,1600,719,971,1249,1375,533,822,1073,1200,0,527.5,853.5,1000,0,388.5,754.4,900,0,5,615.3,800,0,0,532.3,700,0,0,385.6,600,0,0,5,500,0,0,0,400,0,0,0,300,0,0,0,200,0,0,0,175,0,0,0,100,0,0,0,0],4,15)  InterpMethod=Akima spline  InternalRulePriority=Speed  RndMeth=Simplest  InputSameDT=on
  Pump efficiency : Lookup_n-D  NumberOfTableDimensions=1  BreakpointsForDimension1=[0,100,200,300,400,500,600,700,800,900,1000,1075,1200,1300,1375,1600]  Table=[2,15,26,37,46,55,62,67,71,74,75,76,74.5,72,70,50]  InterpMethod=Akima spline  InternalRulePriority=Speed  RndMeth=Simplest  InputSameDT=on
  Rate Transition1 : RateTransition  OutPortSampleTime=0.01
  Rate Transition12 : RateTransition  OutPortSampleTime=0.01
  Rate Transition2 : RateTransition  OutPortSampleTime=0.01
  Saturation : Saturate  UpperLimit=inf  LowerLimit=0
  Simulink-PS Converter1 : nesl_utility/Simulink-PS Converter  PhysicalDomain=network_engine_domain  SubClassName=ps_input  LeftPortType=input  RightPortType=output  PseudoPeriodic=off  Frequencies=[]  NoiseDistribution=none  NoiseParameters=[]  Unit=m^3/s  AffineConversion=off  FilteringAndDerivatives=provide  SimscapeFilterOrder=1  InputFilterTimeConstant=0.001  UdotUserProvided=0
      settings: SourceProductBaseCode=MT,SS
  Subsystem : Subsystem
  output : PMIOPort  Side=Right
  Power : Outport
  wires:
  Gain/1 -> Subsystem/1(flow), Simulink-PS Converter1/1
  Pump characteristic1/1 -> Saturation/1
  Rate Transition2/1 -> ?  "Pump RPM"
  Rate Transition1/1 -> ?  "Pump torque"
  Rate Transition12/1 -> ?  "Pump power"
  Pump efficiency/1 -> Subsystem/2(eff)
  Subsystem/1(Power) -> Power and Flow/2, Power/1, Rate Transition12/1  "Power"
  RPM/1 -> Pump characteristic1/1  "RPM"
  Pump characteristic/1 -> ?
  Pump p/1 -> Pump characteristic1/2, Subsystem/3(p)
  Saturation/1 -> Gain/1, Rate Transition2/1, Power and Flow/1, Pump efficiency/1
  connections:
  output/RConn1 -- Simulink-PS Converter1/RConn1

== system Pump_system_008/Subsystem5/Pump ==
  RPM : Inport
  Pump p : Inport  Port=2
  Gain : Gain  Gain=1/3600
  Power and Flow : Scope  NumInputPorts=2
  Product1 : Product
  Pump characteristic : Lookup_n-D  NumberOfTableDimensions=1  BreakpointsForDimension1=[0,4.4,5.6,7.2,7.8,8.4,8.8,9.3,9.7,10,10.2,10.3,10.35,10.351,10.352]  Table=[1600,1375,1200,1000,900,800,700,600,500,400,300,200,175,100,0]  InterpMethod=Akima spline  InternalRulePriority=Speed  RndMeth=Simplest  InputSameDT=on
  Pump efficiency : Lookup_n-D  NumberOfTableDimensions=1  BreakpointsForDimension1=[0,100,200,300,400,500,600,700,800,900,1000,1075,1200,1300,1375,1600]  Table=[2,15,26,37,46,55,62,67,71,74,75,76,74.5,72,70,50]  InterpMethod=Akima spline  InternalRulePriority=Speed  RndMeth=Simplest  InputSameDT=on
  Rate Transition1 : RateTransition  OutPortSampleTime=1
  Rate Transition12 : RateTransition  OutPortSampleTime=1
  Rate Transition2 : RateTransition  OutPortSampleTime=1
  Simulink-PS Converter1 : nesl_utility/Simulink-PS Converter  PhysicalDomain=network_engine_domain  SubClassName=ps_input  LeftPortType=input  RightPortType=output  PseudoPeriodic=off  Frequencies=[]  NoiseDistribution=none  NoiseParameters=[]  Unit=m^3/s  AffineConversion=off  FilteringAndDerivatives=provide  SimscapeFilterOrder=1  InputFilterTimeConstant=0.001  UdotUserProvided=0
      settings: SourceProductBaseCode=MT,SS
  Subsystem : Subsystem
  output : PMIOPort  Side=Right
  Power : Outport
  wires:
  Gain/1 -> Subsystem/1(flow), Simulink-PS Converter1/1
  Product1/1 -> Gain/1, Rate Transition2/1, Power and Flow/1
  Pump efficiency/1 -> Subsystem/2(eff)
  Subsystem/1(Power) -> Rate Transition12/1, Power and Flow/2, Power/1  "Power"
  Pump p/1 -> Rate Transition1/1, Subsystem/3(p), Pump characteristic/1
  Pump characteristic/1 -> Product1/2, Pump efficiency/1
  RPM/1 -> Product1/1  "RPM"
  Rate Transition12/1 -> ?  "Pump2 power"
  Rate Transition2/1 -> ?  "Pump2 flow"
  Rate Transition1/1 -> ?  "Pump2 pressure"
  connections:
  output/RConn1 -- Simulink-PS Converter1/RConn1

== system Pump_system_008/Subsystem9/Pump ==
  RPM : Inport
  Pump p : Inport  Port=2
  Gain : Gain  Gain=1/3600
  Power and Flow : Scope  NumInputPorts=2
  Product1 : Product
  Pump characteristic : Lookup_n-D  NumberOfTableDimensions=1  BreakpointsForDimension1=[0,4.4,5.6,7.2,7.8,8.4,8.8,9.3,9.7,10,10.2,10.3,10.35,10.351,10.352]  Table=[1600,1375,1200,1000,900,800,700,600,500,400,300,200,175,100,0]  InterpMethod=Akima spline  InternalRulePriority=Speed  RndMeth=Simplest  InputSameDT=on
  Pump efficiency : Lookup_n-D  NumberOfTableDimensions=1  BreakpointsForDimension1=[0,100,200,300,400,500,600,700,800,900,1000,1075,1200,1300,1375,1600]  Table=[2,15,26,37,46,55,62,67,71,74,75,76,74.5,72,70,50]  InterpMethod=Akima spline  InternalRulePriority=Speed  RndMeth=Simplest  InputSameDT=on
  Rate Transition1 : RateTransition  OutPortSampleTime=1
  Rate Transition12 : RateTransition  OutPortSampleTime=1
  Rate Transition2 : RateTransition  OutPortSampleTime=1
  Simulink-PS Converter1 : nesl_utility/Simulink-PS Converter  PhysicalDomain=network_engine_domain  SubClassName=ps_input  LeftPortType=input  RightPortType=output  PseudoPeriodic=off  Frequencies=[]  NoiseDistribution=none  NoiseParameters=[]  Unit=m^3/s  AffineConversion=off  FilteringAndDerivatives=provide  SimscapeFilterOrder=1  InputFilterTimeConstant=0.001  UdotUserProvided=0
      settings: SourceProductBaseCode=MT,SS
  Subsystem : Subsystem
  output : PMIOPort  Side=Right
  Power : Outport
  wires:
  Gain/1 -> Subsystem/1(flow), Simulink-PS Converter1/1
  Product1/1 -> Gain/1, Rate Transition2/1, Power and Flow/1
  Pump efficiency/1 -> Subsystem/2(eff)
  Subsystem/1(Power) -> Rate Transition12/1, Power and Flow/2, Power/1  "Power"
  Pump p/1 -> Rate Transition1/1, Subsystem/3(p), Pump characteristic/1
  Pump characteristic/1 -> Product1/2, Pump efficiency/1
  RPM/1 -> Product1/1  "RPM"
  Rate Transition2/1 -> ?  "Pump3 flow"
  Rate Transition1/1 -> ?  "Pump3 pressure"
  Rate Transition12/1 -> ?  "Pump3 power"
  connections:
  output/RConn1 -- Simulink-PS Converter1/RConn1

== system Pump_system_008/Subsystem12/Pump/Subsystem ==
  flow : Inport
  eff : Inport  Port=2
  p : Inport  Port=3
  Divide1 : Product  Inputs=*/
  Gain1 : Gain  Gain=0.1
  Gain3 : Gain  Gain=10^3
  Gain4 : Gain  Gain=0.01
  Product2 : Product
  Saturation : Saturate  UpperLimit=inf  LowerLimit=208
  Power : Outport
  wires:
  Gain1/1 -> Product2/2
  Product2/1 -> Divide1/1
  flow/1 -> Product2/1
  Divide1/1 -> Gain3/1
  eff/1 -> Gain4/1
  Gain4/1 -> Divide1/2
  p/1 -> Gain1/1
  Gain3/1 -> Saturation/1
  Saturation/1 -> Power/1

== system Pump_system_008/Subsystem21/Pump/Subsystem ==
  flow : Inport
  eff : Inport  Port=2
  p : Inport  Port=3
  Divide1 : Product  Inputs=*/
  Gain1 : Gain  Gain=0.1
  Gain3 : Gain  Gain=10^3
  Gain4 : Gain  Gain=0.01
  Product2 : Product
  Saturation : Saturate  UpperLimit=inf  LowerLimit=10
  Power : Outport
  wires:
  Gain1/1 -> Product2/2
  Product2/1 -> Divide1/1
  flow/1 -> Product2/1
  Divide1/1 -> Gain3/1
  eff/1 -> Gain4/1
  Gain4/1 -> Divide1/2
  p/1 -> Gain1/1
  Gain3/1 -> Saturation/1
  Saturation/1 -> Power/1

== system Pump_system_008/Subsystem25/Pump/Subsystem ==
  flow : Inport
  eff : Inport  Port=2
  p : Inport  Port=3
  Divide1 : Product  Inputs=*/
  Gain1 : Gain  Gain=0.1
  Gain3 : Gain  Gain=10^3
  Gain4 : Gain  Gain=0.01
  Product2 : Product
  Saturation : Saturate  UpperLimit=inf  LowerLimit=208
  Power : Outport
  wires:
  Saturation/1 -> Power/1
  Gain3/1 -> Saturation/1
  p/1 -> Gain1/1
  Gain4/1 -> Divide1/2
  eff/1 -> Gain4/1
  Divide1/1 -> Gain3/1
  flow/1 -> Product2/1
  Product2/1 -> Divide1/1
  Gain1/1 -> Product2/2

== system Pump_system_008/Subsystem5/Pump/Subsystem ==
  flow : Inport
  eff : Inport  Port=2
  p : Inport  Port=3
  Divide1 : Product  Inputs=*/
  Gain1 : Gain  Gain=0.1
  Gain3 : Gain  Gain=10^3
  Gain4 : Gain  Gain=0.01
  Product2 : Product
  Saturation : Saturate  UpperLimit=inf  LowerLimit=208
  Power : Outport
  wires:
  Saturation/1 -> Power/1
  Gain3/1 -> Saturation/1
  p/1 -> Gain1/1
  Gain4/1 -> Divide1/2
  eff/1 -> Gain4/1
  Divide1/1 -> Gain3/1
  flow/1 -> Product2/1
  Product2/1 -> Divide1/1
  Gain1/1 -> Product2/2

== system Pump_system_008/Subsystem9/Pump/Subsystem ==
  flow : Inport
  eff : Inport  Port=2
  p : Inport  Port=3
  Divide1 : Product  Inputs=*/
  Gain1 : Gain  Gain=0.1
  Gain3 : Gain  Gain=10^3
  Gain4 : Gain  Gain=0.01
  Product2 : Product
  Saturation : Saturate  UpperLimit=inf  LowerLimit=208
  Power : Outport
  wires:
  Saturation/1 -> Power/1
  Gain3/1 -> Saturation/1
  p/1 -> Gain1/1
  Gain4/1 -> Divide1/2
  eff/1 -> Gain4/1
  Divide1/1 -> Gain3/1
  flow/1 -> Product2/1
  Product2/1 -> Divide1/1
  Gain1/1 -> Product2/2
